simulink model "SUB_LinControl"  (R2018b)
settings: Solver=VariableStepDiscrete  StartTime=0.0  StopTime=10  RelTol=1e-3
PreLoadFcn:
  | if(exist('MBDS_ModelCallback', 'file'))
  |    MBDS_ModelCallback('PreLoad');
  | end
PostLoadFcn:
  | if(exist('MBDS_ModelCallback', 'file'))
  |    MBDS_ModelCallback('PostLoad');
  | end
InitFcn:
  | if(exist('MBDS_ModelCallback', 'file'))
  |    MBDS_ModelCallback('Init');
  | end
StartFcn:
  | if(exist('MBDS_ModelCallback', 'file'))
  |    MBDS_ModelCallback('Start');
  | end
StopFcn:
  | if(exist('MBDS_ModelCallback', 'file'))
  |    MBDS_ModelCallback('Stop');
  | end
undefined symbols (not defined in the file): sigbuilder_block
libraries: KIBES_Signal x48, simulink x3
(part 2 of 2)

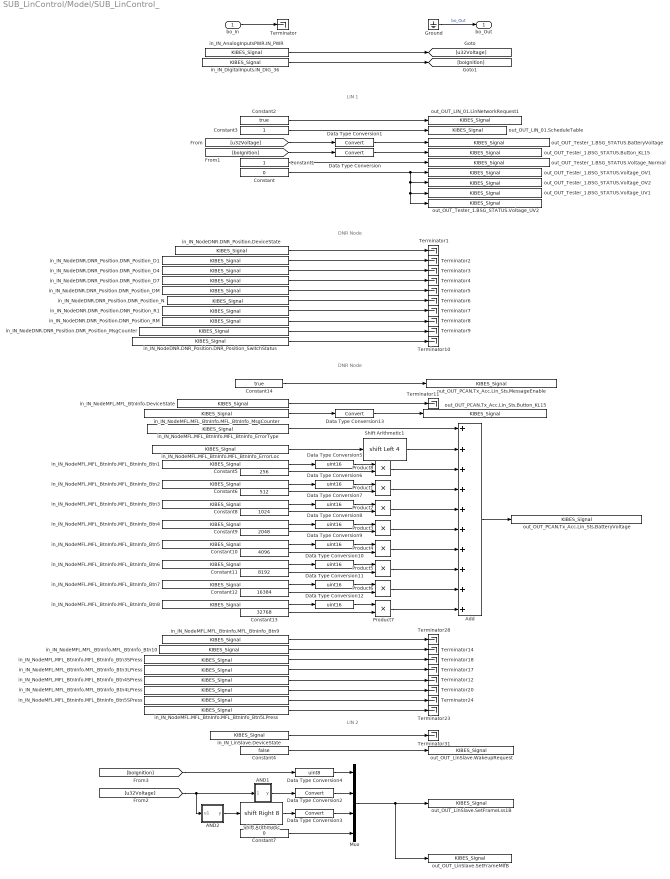
== system SUB_LinControl/Model/SUB_LinControl_ ==
  note: LIN 1
  note: DNR Node
  note: DNR Node
  note: LIN 2
  bo_In : Inport  OutDataTypeStr=boolean
  AND1 : Subsystem  InitFcn=|  mask(AND){MBDS_LibraryBlock=on, BitwiseMode=on, Inputs=1, UseBitMask=on, BitMask='FF', OutDataTypeStr=Inherit: Inherit via back propagation, MBDS_BlockVersion=08.20.02}
      | if(exist('MBDS_BlockCallback', 'file'))
      |    MBDS_BlockCallback('Update', gcb);
      | end
      mask prompts: MBDS_LibraryBlock "MBDS library block"; BitwiseMode "Use 'bitwise' mode"; Inputs "Number of input ports:"; UseBitMask "Use bit mask"; BitMask "Bit mask:"; OutDataTypeStr "Output data type:"; MBDS_BlockVersion "Version:"
      mask help: Logical or bitwise AND operator. For multiple inputs, operators are applied across the inputs. For a single input, operators are applied across the input vector. In bitwise mode a bit mask can be applied onto single input signals.
      mask init:
      | if(exist('MBDS_BlockCallback', 'file'))
      |    MBDS_BlockCallback('Init', gcb);
      | else
      |    % Disable all mask parameters
      |    MaskEnables = get_param(gcb, 'MaskEnables');
      |    for k = [1:length(MaskEnables)]
      |       MaskEnables{k} = 'off';
      |    end
      |    if(~isequal(MaskEnables, get_param(gcb, 'MaskEnables')))
      |       set_param(gcb, 'MaskEnables', MaskEnables);
      |    end
      | end
      settings: AttributesFormatString=bitwise
      mask Help: eval(['open([workdir(''library_dir:''),''\Blockset\help\'',get_param(gcb,''MaskType''),''.html''])'])
      mask Callback BitwiseMode:
      | if(exist('MBDS_BlockCallback', 'file'))
      |    MBDS_BlockCallback('BitwiseMode', gcb);
      | end
      mask Callback Inputs:
      | if(exist('MBDS_BlockCallback', 'file'))
      |    MBDS_BlockCallback('Inputs', gcb);
      | end
      mask Callback UseBitMask:
      | if(exist('MBDS_BlockCallback', 'file'))
      |    MBDS_BlockCallback('UseBitMask', gcb);
      | end
      mask Callback BitMask:
      | if(exist('MBDS_BlockCallback', 'file'))
      |    MBDS_BlockCallback('BitMask', gcb);
      | end
      mask TypeOptions OutDataTypeStr: Inherit: Inherit via back propagation | int8 | uint8 | int16 | uint16 | int32 | uint32 | boolean
      mask Callback OutDataTypeStr:
      | % Adopt Value
      | if(exist('MBDS_BlockCallback', 'file'))
      |    MBDS_BlockCallback('OutDataTypeStr', gcb);
      | end
      mask DialogControl ParameterTabVar0 Prompt: Main
      mask DialogControl ParameterTabVar01 Prompt: Signal Attributes
      mask DialogControl ParameterTabVar012 Prompt: Version
      mask Display:
      | % Show icon or block text
      | if(UseBitMask)
      |    if(isnumeric(BitMask))
      |       BitMaskString = ['0x',dec2hex(floor(BitMask))];
      |    elseif(ischar(BitMask))
      |       BitMaskString = ['0x',upper(BitMask)];
      |    else
      |       BitMaskString = '???';
      |    end
      |    disp(sprintf(['AND\n', BitMaskString]))
      | else
      |    disp('AND')
      | end
  AND2 : Subsystem  InitFcn=|  mask(AND){MBDS_LibraryBlock=on, BitwiseMode=on, Inputs=1, UseBitMask=on, BitMask='FF00', OutDataTypeStr=Inherit: Inherit via back propagation, MBDS_BlockVersion=08.20.02}
      | if(exist('MBDS_BlockCallback', 'file'))
      |    MBDS_BlockCallback('Update', gcb);
      | end
      mask prompts: MBDS_LibraryBlock "MBDS library block"; BitwiseMode "Use 'bitwise' mode"; Inputs "Number of input ports:"; UseBitMask "Use bit mask"; BitMask "Bit mask:"; OutDataTypeStr "Output data type:"; MBDS_BlockVersion "Version:"
      mask help: Logical or bitwise AND operator. For multiple inputs, operators are applied across the inputs. For a single input, operators are applied across the input vector. In bitwise mode a bit mask can be applied onto single input signals.
      mask init: same as SUB_LinControl/Model/SUB_LinControl_/AND1
      settings: AttributesFormatString=bitwise
      mask Help: eval(['open([workdir(''library_dir:''),''\Blockset\help\'',get_param(gcb,''MaskType''),''.html''])'])
      mask Callback BitwiseMode:
      | if(exist('MBDS_BlockCallback', 'file'))
      |    MBDS_BlockCallback('BitwiseMode', gcb);
      | end
      mask Callback Inputs:
      | if(exist('MBDS_BlockCallback', 'file'))
      |    MBDS_BlockCallback('Inputs', gcb);
      | end
      mask Callback UseBitMask:
      | if(exist('MBDS_BlockCallback', 'file'))
      |    MBDS_BlockCallback('UseBitMask', gcb);
      | end
      mask Callback BitMask:
      | if(exist('MBDS_BlockCallback', 'file'))
      |    MBDS_BlockCallback('BitMask', gcb);
      | end
      mask TypeOptions OutDataTypeStr: Inherit: Inherit via back propagation | int8 | uint8 | int16 | uint16 | int32 | uint32 | boolean
      mask Callback OutDataTypeStr:
      | % Adopt Value
      | if(exist('MBDS_BlockCallback', 'file'))
      |    MBDS_BlockCallback('OutDataTypeStr', gcb);
      | end
      mask DialogControl ParameterTabVar0 Prompt: Main
      mask DialogControl ParameterTabVar01 Prompt: Signal Attributes
      mask DialogControl ParameterTabVar012 Prompt: Version
      mask Display:
      | % Show icon or block text
      | if(UseBitMask)
      |    if(isnumeric(BitMask))
      |       BitMaskString = ['0x',dec2hex(floor(BitMask))];
      |    elseif(ischar(BitMask))
      |       BitMaskString = ['0x',upper(BitMask)];
      |    else
      |       BitMaskString = '???';
      |    end
      |    disp(sprintf(['AND\n', BitMaskString]))
      | else
      |    disp('AND')
      | end
  Add : Sum  InitFcn=|  Inputs=++++++++++  AccumDataTypeStr=uint16  OutDataTypeStr=uint16  SaturateOnIntegerOverflow=on
      | if(exist('MBDS_BlockCallback', 'file'))
      |    MBDS_BlockCallback('Update', gcb);  
      | end
      settings: AttributesFormatString=Saturate: %<SaturateOnIntegerOverflow>
  Constant : Constant  InitFcn=|  Value=0  OutDataTypeStr=uint8
      | if(exist('MBDS_BlockCallback', 'file'))
      |    MBDS_BlockCallback('Update', gcb);  
      | end
  Constant1 : Constant  InitFcn=|  OutDataTypeStr=uint8
      | if(exist('MBDS_BlockCallback', 'file'))
      |    MBDS_BlockCallback('Update', gcb);  
      | end
  Constant10 : Constant  InitFcn=|  Value=4096  OutDataTypeStr=uint16
      | if(exist('MBDS_BlockCallback', 'file'))
      |    MBDS_BlockCallback('Update', gcb);  
      | end
  Constant11 : Constant  InitFcn=|  Value=8192  OutDataTypeStr=uint16
      | if(exist('MBDS_BlockCallback', 'file'))
      |    MBDS_BlockCallback('Update', gcb);  
      | end
  Constant12 : Constant  InitFcn=|  Value=16384  OutDataTypeStr=uint16
      | if(exist('MBDS_BlockCallback', 'file'))
      |    MBDS_BlockCallback('Update', gcb);  
      | end
  Constant13 : Constant  InitFcn=|  Value=32768  OutDataTypeStr=uint16
      | if(exist('MBDS_BlockCallback', 'file'))
      |    MBDS_BlockCallback('Update', gcb);  
      | end
  Constant14 : Constant  InitFcn=|  Value=true  OutDataTypeStr=boolean  LockScale=on
      | if(exist('MBDS_BlockCallback', 'file'))
      |    MBDS_BlockCallback('Update', gcb);  
      | end
  Constant2 : Constant  InitFcn=|  Value=true  OutDataTypeStr=boolean
      | if(exist('MBDS_BlockCallback', 'file'))
      |    MBDS_BlockCallback('Update', gcb);  
      | end
  Constant3 : Constant  InitFcn=|  OutDataTypeStr=uint8
      | if(exist('MBDS_BlockCallback', 'file'))
      |    MBDS_BlockCallback('Update', gcb);  
      | end
  Constant4 : Constant  InitFcn=|  Value=false  OutDataTypeStr=boolean
      | if(exist('MBDS_BlockCallback', 'file'))
      |    MBDS_BlockCallback('Update', gcb);  
      | end
  Constant5 : Constant  InitFcn=|  Value=256  OutDataTypeStr=uint16
      | if(exist('MBDS_BlockCallback', 'file'))
      |    MBDS_BlockCallback('Update', gcb);  
      | end
  Constant6 : Constant  InitFcn=|  Value=512  OutDataTypeStr=uint16
      | if(exist('MBDS_BlockCallback', 'file'))
      |    MBDS_BlockCallback('Update', gcb);  
      | end
  Constant7 : Constant  InitFcn=|  Value=0  OutDataTypeStr=uint8
      | if(exist('MBDS_BlockCallback', 'file'))
      |    MBDS_BlockCallback('Update', gcb);  
      | end
  Constant8 : Constant  InitFcn=|  Value=1024  OutDataTypeStr=uint16
      | if(exist('MBDS_BlockCallback', 'file'))
      |    MBDS_BlockCallback('Update', gcb);  
      | end
  Constant9 : Constant  InitFcn=|  Value=2048  OutDataTypeStr=uint16
      | if(exist('MBDS_BlockCallback', 'file'))
      |    MBDS_BlockCallback('Update', gcb);  
      | end
  Data Type Conversion : DataTypeConversion  InitFcn=|  SaturateOnIntegerOverflow=on
      | try
      |    MBDS_BlockCallback('Update', gcb);
      | end
      settings: AttributesFormatString=Saturate: %<SaturateOnIntegerOverflow>
  Data Type Conversion1 : DataTypeConversion  InitFcn=|  SaturateOnIntegerOverflow=on
      | try
      |    MBDS_BlockCallback('Update', gcb);
      | end
      settings: AttributesFormatString=Saturate: %<SaturateOnIntegerOverflow>
  Data Type Conversion10 : DataTypeConversion  InitFcn=|  OutDataTypeStr=uint16  SaturateOnIntegerOverflow=on
      | try
      |    MBDS_BlockCallback('Update', gcb);
      | end
      settings: AttributesFormatString=Saturate: %<SaturateOnIntegerOverflow>
  Data Type Conversion11 : DataTypeConversion  InitFcn=|  OutDataTypeStr=uint16  SaturateOnIntegerOverflow=on
      | try
      |    MBDS_BlockCallback('Update', gcb);
      | end
      settings: AttributesFormatString=Saturate: %<SaturateOnIntegerOverflow>
  Data Type Conversion12 : DataTypeConversion  InitFcn=|  OutDataTypeStr=uint16  SaturateOnIntegerOverflow=on
      | try
      |    MBDS_BlockCallback('Update', gcb);
      | end
      settings: AttributesFormatString=Saturate: %<SaturateOnIntegerOverflow>
  Data Type Conversion13 : DataTypeConversion  InitFcn=|  SaturateOnIntegerOverflow=on
      | try
      |    MBDS_BlockCallback('Update', gcb);
      | end
      settings: AttributesFormatString=Saturate: %<SaturateOnIntegerOverflow>
  Data Type Conversion2 : DataTypeConversion  InitFcn=|
      | try
      |    MBDS_BlockCallback('Update', gcb);
      | end
      settings: AttributesFormatString=Saturate: %<SaturateOnIntegerOverflow>
  Data Type Conversion3 : DataTypeConversion  InitFcn=|
      | try
      |    MBDS_BlockCallback('Update', gcb);
      | end
      settings: AttributesFormatString=Saturate: %<SaturateOnIntegerOverflow>
  Data Type Conversion4 : DataTypeConversion  InitFcn=|  OutDataTypeStr=uint8  SaturateOnIntegerOverflow=on
      | try
      |    MBDS_BlockCallback('Update', gcb);
      | end
      settings: AttributesFormatString=Saturate: %<SaturateOnIntegerOverflow>
  Data Type Conversion5 : DataTypeConversion  InitFcn=|  OutDataTypeStr=uint16  SaturateOnIntegerOverflow=on
      | try
      |    MBDS_BlockCallback('Update', gcb);
      | end
      settings: AttributesFormatString=Saturate: %<SaturateOnIntegerOverflow>
  Data Type Conversion6 : DataTypeConversion  InitFcn=|  OutDataTypeStr=uint16  SaturateOnIntegerOverflow=on
      | try
      |    MBDS_BlockCallback('Update', gcb);
      | end
      settings: AttributesFormatString=Saturate: %<SaturateOnIntegerOverflow>
  Data Type Conversion7 : DataTypeConversion  InitFcn=|  OutDataTypeStr=uint16  SaturateOnIntegerOverflow=on
      | try
      |    MBDS_BlockCallback('Update', gcb);
      | end
      settings: AttributesFormatString=Saturate: %<SaturateOnIntegerOverflow>
  Data Type Conversion8 : DataTypeConversion  InitFcn=|  OutDataTypeStr=uint16  SaturateOnIntegerOverflow=on
      | try
      |    MBDS_BlockCallback('Update', gcb);
      | end
      settings: AttributesFormatString=Saturate: %<SaturateOnIntegerOverflow>
  Data Type Conversion9 : DataTypeConversion  InitFcn=|  OutDataTypeStr=uint16  SaturateOnIntegerOverflow=on
      | try
      |    MBDS_BlockCallback('Update', gcb);
      | end
      settings: AttributesFormatString=Saturate: %<SaturateOnIntegerOverflow>
  Ground : Ground  InitFcn=|
      | try
      |    MBDS_BlockCallback('Update', gcb);
      | end
      settings: MoveFcn=UpdateBlockSize(gcb);
  Mux : Mux  InitFcn=|
      | try
      |    MBDS_BlockCallback('Update', gcb);
      | end
  Product1 : Product  InitFcn=|  Inputs=**  OutDataTypeStr=uint16  SaturateOnIntegerOverflow=on
      | if(exist('MBDS_BlockCallback', 'file'))
      |    MBDS_BlockCallback('Update', gcb);  
      | end
      settings: AttributesFormatString=Saturate: %<SaturateOnIntegerOverflow>
  Product2 : Product  InitFcn=|  Inputs=**  OutDataTypeStr=uint16  SaturateOnIntegerOverflow=on
      | if(exist('MBDS_BlockCallback', 'file'))
      |    MBDS_BlockCallback('Update', gcb);  
      | end
      settings: AttributesFormatString=Saturate: %<SaturateOnIntegerOverflow>
  Product3 : Product  InitFcn=|  Inputs=**  OutDataTypeStr=uint16  SaturateOnIntegerOverflow=on
      | if(exist('MBDS_BlockCallback', 'file'))
      |    MBDS_BlockCallback('Update', gcb);  
      | end
      settings: AttributesFormatString=Saturate: %<SaturateOnIntegerOverflow>
  Product4 : Product  InitFcn=|  Inputs=**  OutDataTypeStr=uint16  SaturateOnIntegerOverflow=on
      | if(exist('MBDS_BlockCallback', 'file'))
      |    MBDS_BlockCallback('Update', gcb);  
      | end
      settings: AttributesFormatString=Saturate: %<SaturateOnIntegerOverflow>
  Product5 : Product  InitFcn=|  Inputs=**  OutDataTypeStr=uint16  SaturateOnIntegerOverflow=on
      | if(exist('MBDS_BlockCallback', 'file'))
      |    MBDS_BlockCallback('Update', gcb);  
      | end
      settings: AttributesFormatString=Saturate: %<SaturateOnIntegerOverflow>
  Product6 : Product  InitFcn=|  Inputs=**  OutDataTypeStr=uint16  SaturateOnIntegerOverflow=on
      | if(exist('MBDS_BlockCallback', 'file'))
      |    MBDS_BlockCallback('Update', gcb);  
      | end
      settings: AttributesFormatString=Saturate: %<SaturateOnIntegerOverflow>
  Product7 : Product  InitFcn=|  Inputs=**  OutDataTypeStr=uint16  SaturateOnIntegerOverflow=on
      | if(exist('MBDS_BlockCallback', 'file'))
      |    MBDS_BlockCallback('Update', gcb);  
      | end
      settings: AttributesFormatString=Saturate: %<SaturateOnIntegerOverflow>
  Product8 : Product  InitFcn=|  Inputs=**  OutDataTypeStr=uint16  SaturateOnIntegerOverflow=on
      | if(exist('MBDS_BlockCallback', 'file'))
      |    MBDS_BlockCallback('Update', gcb);  
      | end
      settings: AttributesFormatString=Saturate: %<SaturateOnIntegerOverflow>
  Shift Arithmetic : ArithShift  InitFcn=|  BitShiftNumber=8  BitShiftDirection=Right
      | try
      |    MBDS_BlockCallback('Update', gcb);
      | end
  Shift Arithmetic1 : ArithShift  InitFcn=|  BitShiftNumber=4  BitShiftDirection=Left
      | try
      |    MBDS_BlockCallback('Update', gcb);
      | end
  Terminator{,1..12,14,17..18,20,23..24,28,31} (21 alike) : Terminator
      settings: MoveFcn=UpdateBlockSize(gcb);
      settings: InitFcn=|
      | try
      |    MBDS_BlockCallback('Update', gcb);
      | end
  in_IN_AnalogInputsPWR.IN_PWR : KIBES_Signal/KIBES_Signal  MBDS_LibraryBlock=on  DatabaseKey=721  SignalName=IN_AnalogInputsPWR.IN_PWR  SymbolName=IN_AnalogInputsPWR_IN_PWR_000721  DataType=uint32  Init=0  Slope=1  Bias=0  DataSize=1  fpDataType=uint32  BlockIOType=Inport  DeviceType=0
  in_IN_DigitalInputs.IN_DIG_36 : KIBES_Signal/KIBES_Signal  MBDS_LibraryBlock=on  DatabaseKey=60  SignalName=IN_DigitalInputs.IN_DIG_36  SymbolName=IN_DigitalInputs_IN_DIG_36_000060  DataType=boolean  Init=0  Slope=1  Bias=0  DataSize=1  fpDataType=boolean  BlockIOType=Inport  DeviceType=0
  in_IN_LinSlave.DeviceState : KIBES_Signal/KIBES_Signal  MBDS_LibraryBlock=on  DatabaseKey=2325  SignalName=IN_LinSlave.DeviceState  SymbolName=IN_LinSlave_DeviceState_002325  DataType=uint16  Init=0  Slope=1  Bias=0  DataSize=1  fpDataType=uint16  BlockIOType=Inport  DeviceType=0
  in_IN_NodeDNR.DNR_Position.DNR_Position_D1 : KIBES_Signal/KIBES_Signal  MBDS_LibraryBlock=on  DatabaseKey=1352  SignalName=IN_NodeDNR.DNR_Position.DNR_Position_D1  SymbolName=IN_NodeDNR_DNR_Position_DNR_Position_D1_001352  DataType=uint8  Init=0  Slope=1  Bias=0  DataSize=1  fpDataType=uint8  BlockIOType=Inport  DeviceType=0
  in_IN_NodeDNR.DNR_Position.DNR_Position_D4 : KIBES_Signal/KIBES_Signal  MBDS_LibraryBlock=on  DatabaseKey=1353  SignalName=IN_NodeDNR.DNR_Position.DNR_Position_D4  SymbolName=IN_NodeDNR_DNR_Position_DNR_Position_D4_001353  DataType=uint8  Init=0  Slope=1  Bias=0  DataSize=1  fpDataType=uint8  BlockIOType=Inport  DeviceType=0
  in_IN_NodeDNR.DNR_Position.DNR_Position_D7 : KIBES_Signal/KIBES_Signal  MBDS_LibraryBlock=on  DatabaseKey=1354  SignalName=IN_NodeDNR.DNR_Position.DNR_Position_D7  SymbolName=IN_NodeDNR_DNR_Position_DNR_Position_D7_001354  DataType=uint8  Init=0  Slope=1  Bias=0  DataSize=1  fpDataType=uint8  BlockIOType=Inport  DeviceType=0
  in_IN_NodeDNR.DNR_Position.DNR_Position_DM : KIBES_Signal/KIBES_Signal  MBDS_LibraryBlock=on  DatabaseKey=1355  SignalName=IN_NodeDNR.DNR_Position.DNR_Position_DM  SymbolName=IN_NodeDNR_DNR_Position_DNR_Position_DM_001355  DataType=uint8  Init=0  Slope=1  Bias=0  DataSize=1  fpDataType=uint8  BlockIOType=Inport  DeviceType=0
  in_IN_NodeDNR.DNR_Position.DNR_Position_MsgCounter : KIBES_Signal/KIBES_Signal  MBDS_LibraryBlock=on  DatabaseKey=1356  SignalName=IN_NodeDNR.DNR_Position.DNR_Position_MsgCounter  SymbolName=IN_NodeDNR_DNR_Position_DNR_Position_MsgCounter_001356  DataType=uint8  Init=0  Slope=1  Bias=0  DataSize=1  fpDataType=uint8  BlockIOType=Inport  DeviceType=0
  in_IN_NodeDNR.DNR_Position.DNR_Position_N : KIBES_Signal/KIBES_Signal  MBDS_LibraryBlock=on  DatabaseKey=1351  SignalName=IN_NodeDNR.DNR_Position.DNR_Position_N  SymbolName=IN_NodeDNR_DNR_Position_DNR_Position_N_001351  DataType=uint8  Init=0  Slope=1  Bias=0  DataSize=1  fpDataType=uint8  BlockIOType=Inport  DeviceType=0
  in_IN_NodeDNR.DNR_Position.DNR_Position_R1 : KIBES_Signal/KIBES_Signal  MBDS_LibraryBlock=on  DatabaseKey=1350  SignalName=IN_NodeDNR.DNR_Position.DNR_Position_R1  SymbolName=IN_NodeDNR_DNR_Position_DNR_Position_R1_001350  DataType=uint8  Init=0  Slope=1  Bias=0  DataSize=1  fpDataType=uint8  BlockIOType=Inport  DeviceType=0
  in_IN_NodeDNR.DNR_Position.DNR_Position_RM : KIBES_Signal/KIBES_Signal  MBDS_LibraryBlock=on  DatabaseKey=1349  SignalName=IN_NodeDNR.DNR_Position.DNR_Position_RM  SymbolName=IN_NodeDNR_DNR_Position_DNR_Position_RM_001349  DataType=uint8  Init=0  Slope=1  Bias=0  DataSize=1  fpDataType=uint8  BlockIOType=Inport  DeviceType=0
  in_IN_NodeDNR.DNR_Position.DNR_Position_SwitchStatus : KIBES_Signal/KIBES_Signal  MBDS_LibraryBlock=on  DatabaseKey=1357  SignalName=IN_NodeDNR.DNR_Position.DNR_Position_SwitchStatus  SymbolName=IN_NodeDNR_DNR_Position_DNR_Position_SwitchStatus_001357  DataType=uint8  Init=0  Slope=1  Bias=0  DataSize=1  fpDataType=uint8  BlockIOType=Inport  DeviceType=0
  in_IN_NodeDNR.DNR_Position.DeviceState : KIBES_Signal/KIBES_Signal  MBDS_LibraryBlock=on  DatabaseKey=2273  SignalName=IN_NodeDNR.DNR_Position.DeviceState  SymbolName=IN_NodeDNR_DNR_Position_DeviceState_002273  DataType=uint16  Init=0  Slope=1  Bias=0  DataSize=1  fpDataType=uint16  BlockIOType=Inport  DeviceType=0
  in_IN_NodeMFL.MFL_BtnInfo.DeviceState : KIBES_Signal/KIBES_Signal  MBDS_LibraryBlock=on  DatabaseKey=2272  SignalName=IN_NodeMFL.MFL_BtnInfo.DeviceState  SymbolName=IN_NodeMFL_MFL_BtnInfo_DeviceState_002272  DataType=uint16  Init=0  Slope=1  Bias=0  DataSize=1  fpDataType=uint16  BlockIOType=Inport  DeviceType=0
  in_IN_NodeMFL.MFL_BtnInfo.MFL_BtnInfo_Btn1 : KIBES_Signal/KIBES_Signal  MBDS_LibraryBlock=on  DatabaseKey=1361  SignalName=IN_NodeMFL.MFL_BtnInfo.MFL_BtnInfo_Btn1  SymbolName=IN_NodeMFL_MFL_BtnInfo_MFL_BtnInfo_Btn1_001361  DataType=uint8  Init=0  Slope=1  Bias=0  DataSize=1  fpDataType=uint8  BlockIOType=Inport  DeviceType=0
  in_IN_NodeMFL.MFL_BtnInfo.MFL_BtnInfo_Btn10 : KIBES_Signal/KIBES_Signal  MBDS_LibraryBlock=on  DatabaseKey=1370  SignalName=IN_NodeMFL.MFL_BtnInfo.MFL_BtnInfo_Btn10  SymbolName=IN_NodeMFL_MFL_BtnInfo_MFL_BtnInfo_Btn10_001370  DataType=uint8  Init=0  Slope=1  Bias=0  DataSize=1  fpDataType=uint8  BlockIOType=Inport  DeviceType=0
  in_IN_NodeMFL.MFL_BtnInfo.MFL_BtnInfo_Btn2 : KIBES_Signal/KIBES_Signal  MBDS_LibraryBlock=on  DatabaseKey=1362  SignalName=IN_NodeMFL.MFL_BtnInfo.MFL_BtnInfo_Btn2  SymbolName=IN_NodeMFL_MFL_BtnInfo_MFL_BtnInfo_Btn2_001362  DataType=uint8  Init=0  Slope=1  Bias=0  DataSize=1  fpDataType=uint8  BlockIOType=Inport  DeviceType=0
  in_IN_NodeMFL.MFL_BtnInfo.MFL_BtnInfo_Btn3 : KIBES_Signal/KIBES_Signal  MBDS_LibraryBlock=on  DatabaseKey=1363  SignalName=IN_NodeMFL.MFL_BtnInfo.MFL_BtnInfo_Btn3  SymbolName=IN_NodeMFL_MFL_BtnInfo_MFL_BtnInfo_Btn3_001363  DataType=uint8  Init=0  Slope=1  Bias=0  DataSize=1  fpDataType=uint8  BlockIOType=Inport  DeviceType=0
  in_IN_NodeMFL.MFL_BtnInfo.MFL_BtnInfo_Btn3LPress : KIBES_Signal/KIBES_Signal  MBDS_LibraryBlock=on  DatabaseKey=1372  SignalName=IN_NodeMFL.MFL_BtnInfo.MFL_BtnInfo_Btn3LPress  SymbolName=IN_NodeMFL_MFL_BtnInfo_MFL_BtnInfo_Btn3LPress_001372  DataType=uint8  Init=0  Slope=1  Bias=0  DataSize=1  fpDataType=uint8  BlockIOType=Inport  DeviceType=0
  in_IN_NodeMFL.MFL_BtnInfo.MFL_BtnInfo_Btn3SPress : KIBES_Signal/KIBES_Signal  MBDS_LibraryBlock=on  DatabaseKey=1371  SignalName=IN_NodeMFL.MFL_BtnInfo.MFL_BtnInfo_Btn3SPress  SymbolName=IN_NodeMFL_MFL_BtnInfo_MFL_BtnInfo_Btn3SPress_001371  DataType=uint8  Init=0  Slope=1  Bias=0  DataSize=1  fpDataType=uint8  BlockIOType=Inport  DeviceType=0
  in_IN_NodeMFL.MFL_BtnInfo.MFL_BtnInfo_Btn4 : KIBES_Signal/KIBES_Signal  MBDS_LibraryBlock=on  DatabaseKey=1364  SignalName=IN_NodeMFL.MFL_BtnInfo.MFL_BtnInfo_Btn4  SymbolName=IN_NodeMFL_MFL_BtnInfo_MFL_BtnInfo_Btn4_001364  DataType=uint8  Init=0  Slope=1  Bias=0  DataSize=1  fpDataType=uint8  BlockIOType=Inport  DeviceType=0
  in_IN_NodeMFL.MFL_BtnInfo.MFL_BtnInfo_Btn4LPress : KIBES_Signal/KIBES_Signal  MBDS_LibraryBlock=on  DatabaseKey=1374  SignalName=IN_NodeMFL.MFL_BtnInfo.MFL_BtnInfo_Btn4LPress  SymbolName=IN_NodeMFL_MFL_BtnInfo_MFL_BtnInfo_Btn4LPress_001374  DataType=uint8  Init=0  Slope=1  Bias=0  DataSize=1  fpDataType=uint8  BlockIOType=Inport  DeviceType=0
  in_IN_NodeMFL.MFL_BtnInfo.MFL_BtnInfo_Btn4SPress : KIBES_Signal/KIBES_Signal  MBDS_LibraryBlock=on  DatabaseKey=1373  SignalName=IN_NodeMFL.MFL_BtnInfo.MFL_BtnInfo_Btn4SPress  SymbolName=IN_NodeMFL_MFL_BtnInfo_MFL_BtnInfo_Btn4SPress_001373  DataType=uint8  Init=0  Slope=1  Bias=0  DataSize=1  fpDataType=uint8  BlockIOType=Inport  DeviceType=0
  in_IN_NodeMFL.MFL_BtnInfo.MFL_BtnInfo_Btn5 : KIBES_Signal/KIBES_Signal  MBDS_LibraryBlock=on  DatabaseKey=1365  SignalName=IN_NodeMFL.MFL_BtnInfo.MFL_BtnInfo_Btn5  SymbolName=IN_NodeMFL_MFL_BtnInfo_MFL_BtnInfo_Btn5_001365  DataType=uint8  Init=0  Slope=1  Bias=0  DataSize=1  fpDataType=uint8  BlockIOType=Inport  DeviceType=0
  in_IN_NodeMFL.MFL_BtnInfo.MFL_BtnInfo_Btn5LPress : KIBES_Signal/KIBES_Signal  MBDS_LibraryBlock=on  DatabaseKey=1376  SignalName=IN_NodeMFL.MFL_BtnInfo.MFL_BtnInfo_Btn5LPress  SymbolName=IN_NodeMFL_MFL_BtnInfo_MFL_BtnInfo_Btn5LPress_001376  DataType=uint8  Init=0  Slope=1  Bias=0  DataSize=1  fpDataType=uint8  BlockIOType=Inport  DeviceType=0
  in_IN_NodeMFL.MFL_BtnInfo.MFL_BtnInfo_Btn5SPress : KIBES_Signal/KIBES_Signal  MBDS_LibraryBlock=on  DatabaseKey=1375  SignalName=IN_NodeMFL.MFL_BtnInfo.MFL_BtnInfo_Btn5SPress  SymbolName=IN_NodeMFL_MFL_BtnInfo_MFL_BtnInfo_Btn5SPress_001375  DataType=uint8  Init=0  Slope=1  Bias=0  DataSize=1  fpDataType=uint8  BlockIOType=Inport  DeviceType=0
  in_IN_NodeMFL.MFL_BtnInfo.MFL_BtnInfo_Btn6 : KIBES_Signal/KIBES_Signal  MBDS_LibraryBlock=on  DatabaseKey=1366  SignalName=IN_NodeMFL.MFL_BtnInfo.MFL_BtnInfo_Btn6  SymbolName=IN_NodeMFL_MFL_BtnInfo_MFL_BtnInfo_Btn6_001366  DataType=uint8  Init=0  Slope=1  Bias=0  DataSize=1  fpDataType=uint8  BlockIOType=Inport  DeviceType=0
  in_IN_NodeMFL.MFL_BtnInfo.MFL_BtnInfo_Btn7 : KIBES_Signal/KIBES_Signal  MBDS_LibraryBlock=on  DatabaseKey=1367  SignalName=IN_NodeMFL.MFL_BtnInfo.MFL_BtnInfo_Btn7  SymbolName=IN_NodeMFL_MFL_BtnInfo_MFL_BtnInfo_Btn7_001367  DataType=uint8  Init=0  Slope=1  Bias=0  DataSize=1  fpDataType=uint8  BlockIOType=Inport  DeviceType=0
  in_IN_NodeMFL.MFL_BtnInfo.MFL_BtnInfo_Btn8 : KIBES_Signal/KIBES_Signal  MBDS_LibraryBlock=on  DatabaseKey=1368  SignalName=IN_NodeMFL.MFL_BtnInfo.MFL_BtnInfo_Btn8  SymbolName=IN_NodeMFL_MFL_BtnInfo_MFL_BtnInfo_Btn8_001368  DataType=uint8  Init=0  Slope=1  Bias=0  DataSize=1  fpDataType=uint8  BlockIOType=Inport  DeviceType=0
  in_IN_NodeMFL.MFL_BtnInfo.MFL_BtnInfo_Btn9 : KIBES_Signal/KIBES_Signal  MBDS_LibraryBlock=on  DatabaseKey=1369  SignalName=IN_NodeMFL.MFL_BtnInfo.MFL_BtnInfo_Btn9  SymbolName=IN_NodeMFL_MFL_BtnInfo_MFL_BtnInfo_Btn9_001369  DataType=uint8  Init=0  Slope=1  Bias=0  DataSize=1  fpDataType=uint8  BlockIOType=Inport  DeviceType=0
  in_IN_NodeMFL.MFL_BtnInfo.MFL_BtnInfo_ErrorLoc : KIBES_Signal/KIBES_Signal  MBDS_LibraryBlock=on  DatabaseKey=1360  SignalName=IN_NodeMFL.MFL_BtnInfo.MFL_BtnInfo_ErrorLoc  SymbolName=IN_NodeMFL_MFL_BtnInfo_MFL_BtnInfo_ErrorLoc_001360  DataType=uint8  Init=0  Slope=1  Bias=0  DataSize=1  fpDataType=uint8  BlockIOType=Inport  DeviceType=0
  in_IN_NodeMFL.MFL_BtnInfo.MFL_BtnInfo_ErrorType : KIBES_Signal/KIBES_Signal  MBDS_LibraryBlock=on  DatabaseKey=1359  SignalName=IN_NodeMFL.MFL_BtnInfo.MFL_BtnInfo_ErrorType  SymbolName=IN_NodeMFL_MFL_BtnInfo_MFL_BtnInfo_ErrorType_001359  DataType=uint8  Init=0  Slope=1  Bias=0  DataSize=1  fpDataType=uint8  BlockIOType=Inport  DeviceType=0
  in_IN_NodeMFL.MFL_BtnInfo.MFL_BtnInfo_MsgCounter : KIBES_Signal/KIBES_Signal  MBDS_LibraryBlock=on  DatabaseKey=1358  SignalName=IN_NodeMFL.MFL_BtnInfo.MFL_BtnInfo_MsgCounter  SymbolName=IN_NodeMFL_MFL_BtnInfo_MFL_BtnInfo_MsgCounter_001358  DataType=uint8  Init=0  Slope=1  Bias=0  DataSize=1  fpDataType=uint8  BlockIOType=Inport  DeviceType=0
  out_OUT_LIN_01.LinNetworkRequest1 : KIBES_Signal/KIBES_Signal  MBDS_LibraryBlock=on  DatabaseKey=1396  SignalName=OUT_LIN_01.LinNetworkRequest1  SymbolName=OUT_LIN_01_LinNetworkRequest1_001396  DataType=boolean  Init=0  Slope=1  Bias=0  DataSize=1  fpDataType=boolean  BlockIOType=Outport  DeviceType=0
  out_OUT_LIN_01.ScheduleTable : KIBES_Signal/KIBES_Signal  MBDS_LibraryBlock=on  DatabaseKey=1397  SignalName=OUT_LIN_01.ScheduleTable  SymbolName=OUT_LIN_01_ScheduleTable_001397  DataType=uint8  Init=0  Slope=1  Bias=0  DataSize=1  fpDataType=uint8  BlockIOType=Outport  DeviceType=0
  out_OUT_LinSlave.SetFrameLss1B : KIBES_Signal/KIBES_Signal  MBDS_LibraryBlock=on  DatabaseKey=2326  SignalName=OUT_LinSlave.SetFrameLss1B  SymbolName=OUT_LinSlave_SetFrameLss1B_002326  DataType=uint8  Init=[0 0 0 0]  Slope=1  Bias=0  DataSize=4  fpDataType=uint8  BlockIOType=Outport  DeviceType=0
  out_OUT_LinSlave.SetFrameMlfB : KIBES_Signal/KIBES_Signal  MBDS_LibraryBlock=on  DatabaseKey=2327  SignalName=OUT_LinSlave.SetFrameMlfB  SymbolName=OUT_LinSlave_SetFrameMlfB_002327  DataType=uint8  Init=[0 0 0 0]  Slope=1  Bias=0  DataSize=4  fpDataType=uint8  BlockIOType=Outport  DeviceType=0
  out_OUT_LinSlave.WakeupRequest : KIBES_Signal/KIBES_Signal  MBDS_LibraryBlock=on  DatabaseKey=2328  SignalName=OUT_LinSlave.WakeupRequest  SymbolName=OUT_LinSlave_WakeupRequest_002328  DataType=boolean  Init=0  Slope=1  Bias=0  DataSize=1  fpDataType=boolean  BlockIOType=Outport  DeviceType=0
  out_OUT_PCAN.Tx_Acc.Lin_Sts.BatteryVoltage : KIBES_Signal/KIBES_Signal  MBDS_LibraryBlock=on  DatabaseKey=1647  SignalName=OUT_PCAN.Tx_Acc.Lin_Sts.BatteryVoltage  SymbolName=OUT_PCAN_Tx_Acc_Lin_Sts_BatteryVoltage_001647  DataType=uint16  Init=0  Slope=1  Bias=0  DataSize=1  fpDataType=uint16  BlockIOType=Outport  DeviceType=0
  out_OUT_PCAN.Tx_Acc.Lin_Sts.Button_KL15 : KIBES_Signal/KIBES_Signal  MBDS_LibraryBlock=on  DatabaseKey=1648  SignalName=OUT_PCAN.Tx_Acc.Lin_Sts.Button_KL15  SymbolName=OUT_PCAN_Tx_Acc_Lin_Sts_Button_KL15_001648  DataType=boolean  Init=0  Slope=1  Bias=0  DataSize=1  fpDataType=boolean  BlockIOType=Outport  DeviceType=0
  out_OUT_PCAN.Tx_Acc.Lin_Sts.MessageEnable : KIBES_Signal/KIBES_Signal  MBDS_LibraryBlock=on  DatabaseKey=1677  SignalName=OUT_PCAN.Tx_Acc.Lin_Sts.MessageEnable  SymbolName=OUT_PCAN_Tx_Acc_Lin_Sts_MessageEnable_001677  DataType=boolean  Init=0  Slope=1  Bias=0  DataSize=1  fpDataType=boolean  BlockIOType=Outport  DeviceType=0
  out_OUT_Tester_1.BSG_STATUS.BatteryVoltage : KIBES_Signal/KIBES_Signal  MBDS_LibraryBlock=on  DatabaseKey=1395  SignalName=OUT_Tester_1.BSG_STATUS.BatteryVoltage  SymbolName=OUT_Tester_1_BSG_STATUS_BatteryVoltage_001395  DataType=uint16  Init=0  Slope=1  Bias=0  DataSize=1  fpDataType=uint16  BlockIOType=Outport  DeviceType=0
  out_OUT_Tester_1.BSG_STATUS.Button_KL15 : KIBES_Signal/KIBES_Signal  MBDS_LibraryBlock=on  DatabaseKey=1389  SignalName=OUT_Tester_1.BSG_STATUS.Button_KL15  SymbolName=OUT_Tester_1_BSG_STATUS_Button_KL15_001389  DataType=uint8  Init=0  Slope=1  Bias=0  DataSize=1  fpDataType=uint8  BlockIOType=Outport  DeviceType=0
  out_OUT_Tester_1.BSG_STATUS.Voltage_Normal : KIBES_Signal/KIBES_Signal  MBDS_LibraryBlock=on  DatabaseKey=1390  SignalName=OUT_Tester_1.BSG_STATUS.Voltage_Normal  SymbolName=OUT_Tester_1_BSG_STATUS_Voltage_Normal_001390  DataType=uint8  Init=0  Slope=1  Bias=0  DataSize=1  fpDataType=uint8  BlockIOType=Outport  DeviceType=0
  out_OUT_Tester_1.BSG_STATUS.Voltage_OV1 : KIBES_Signal/KIBES_Signal  MBDS_LibraryBlock=on  DatabaseKey=1391  SignalName=OUT_Tester_1.BSG_STATUS.Voltage_OV1  SymbolName=OUT_Tester_1_BSG_STATUS_Voltage_OV1_001391  DataType=uint8  Init=0  Slope=1  Bias=0  DataSize=1  fpDataType=uint8  BlockIOType=Outport  DeviceType=0
  out_OUT_Tester_1.BSG_STATUS.Voltage_OV2 : KIBES_Signal/KIBES_Signal  MBDS_LibraryBlock=on  DatabaseKey=1392  SignalName=OUT_Tester_1.BSG_STATUS.Voltage_OV2  SymbolName=OUT_Tester_1_BSG_STATUS_Voltage_OV2_001392  DataType=uint8  Init=0  Slope=1  Bias=0  DataSize=1  fpDataType=uint8  BlockIOType=Outport  DeviceType=0
  out_OUT_Tester_1.BSG_STATUS.Voltage_UV1 : KIBES_Signal/KIBES_Signal  MBDS_LibraryBlock=on  DatabaseKey=1393  SignalName=OUT_Tester_1.BSG_STATUS.Voltage_UV1  SymbolName=OUT_Tester_1_BSG_STATUS_Voltage_UV1_001393  DataType=uint8  Init=0  Slope=1  Bias=0  DataSize=1  fpDataType=uint8  BlockIOType=Outport  DeviceType=0
  out_OUT_Tester_1.BSG_STATUS.Voltage_UV2 : KIBES_Signal/KIBES_Signal  MBDS_LibraryBlock=on  DatabaseKey=1394  SignalName=OUT_Tester_1.BSG_STATUS.Voltage_UV2  SymbolName=OUT_Tester_1_BSG_STATUS_Voltage_UV2_001394  DataType=uint8  Init=0  Slope=1  Bias=0  DataSize=1  fpDataType=uint8  BlockIOType=Outport  DeviceType=0
  bo_Out : Outport  OutDataTypeStr=boolean
  wires:
  bo_In/1 -> Terminator/1
  Ground/1 -> bo_Out/1  "bo_Out"
  Constant/1 -> out_OUT_Tester_1.BSG_STATUS.Voltage_UV2/1, out_OUT_Tester_1.BSG_STATUS.Voltage_UV1/1, out_OUT_Tester_1.BSG_STATUS.Voltage_OV2/1, out_OUT_Tester_1.BSG_STATUS.Voltage_OV1/1
  Constant1/1 -> out_OUT_Tester_1.BSG_STATUS.Voltage_Normal/1
  [boIgnition] -> Data Type Conversion/1
  Data Type Conversion/1 -> out_OUT_Tester_1.BSG_STATUS.Button_KL15/1
  [u32Voltage] -> Data Type Conversion1/1
  Data Type Conversion1/1 -> out_OUT_Tester_1.BSG_STATUS.BatteryVoltage/1
  Constant2/1 -> out_OUT_LIN_01.LinNetworkRequest1/1
  Constant3/1 -> out_OUT_LIN_01.ScheduleTable/1
  in_IN_NodeDNR.DNR_Position.DeviceState/1 -> Terminator1/1
  in_IN_NodeDNR.DNR_Position.DNR_Position_D1/1 -> Terminator2/1
  in_IN_NodeDNR.DNR_Position.DNR_Position_D4/1 -> Terminator3/1
  in_IN_NodeDNR.DNR_Position.DNR_Position_D7/1 -> Terminator4/1
  in_IN_NodeDNR.DNR_Position.DNR_Position_DM/1 -> Terminator5/1
  in_IN_NodeDNR.DNR_Position.DNR_Position_N/1 -> Terminator6/1
  in_IN_NodeDNR.DNR_Position.DNR_Position_R1/1 -> Terminator7/1
  in_IN_NodeDNR.DNR_Position.DNR_Position_RM/1 -> Terminator8/1
  in_IN_NodeDNR.DNR_Position.DNR_Position_MsgCounter/1 -> Terminator9/1
  in_IN_NodeDNR.DNR_Position.DNR_Position_SwitchStatus/1 -> Terminator10/1
  in_IN_NodeMFL.MFL_BtnInfo.DeviceState/1 -> Terminator11/1
  in_IN_NodeMFL.MFL_BtnInfo.MFL_BtnInfo_Btn1/1 -> Data Type Conversion5/1
  in_IN_NodeMFL.MFL_BtnInfo.MFL_BtnInfo_Btn10/1 -> Terminator14/1
  in_IN_NodeMFL.MFL_BtnInfo.MFL_BtnInfo_Btn2/1 -> Data Type Conversion6/1
  in_IN_NodeMFL.MFL_BtnInfo.MFL_BtnInfo_Btn3/1 -> Data Type Conversion7/1
  in_IN_NodeMFL.MFL_BtnInfo.MFL_BtnInfo_Btn3LPress/1 -> Terminator17/1
  in_IN_NodeMFL.MFL_BtnInfo.MFL_BtnInfo_Btn3SPress/1 -> Terminator18/1
  in_IN_NodeMFL.MFL_BtnInfo.MFL_BtnInfo_Btn4/1 -> Data Type Conversion8/1
  in_IN_NodeMFL.MFL_BtnInfo.MFL_BtnInfo_Btn4LPress/1 -> Terminator20/1
  in_IN_NodeMFL.MFL_BtnInfo.MFL_BtnInfo_Btn4SPress/1 -> Terminator12/1
  in_IN_NodeMFL.MFL_BtnInfo.MFL_BtnInfo_Btn5/1 -> Data Type Conversion9/1
  in_IN_NodeMFL.MFL_BtnInfo.MFL_BtnInfo_Btn5LPress/1 -> Terminator23/1
  in_IN_NodeMFL.MFL_BtnInfo.MFL_BtnInfo_Btn5SPress/1 -> Terminator24/1
  in_IN_NodeMFL.MFL_BtnInfo.MFL_BtnInfo_Btn6/1 -> Data Type Conversion10/1
  in_IN_NodeMFL.MFL_BtnInfo.MFL_BtnInfo_Btn7/1 -> Data Type Conversion11/1
  in_IN_NodeMFL.MFL_BtnInfo.MFL_BtnInfo_Btn8/1 -> Data Type Conversion12/1
  in_IN_NodeMFL.MFL_BtnInfo.MFL_BtnInfo_Btn9/1 -> Terminator28/1
  in_IN_NodeMFL.MFL_BtnInfo.MFL_BtnInfo_ErrorLoc/1 -> Shift Arithmetic1/1
  in_IN_NodeMFL.MFL_BtnInfo.MFL_BtnInfo_ErrorType/1 -> Add/1
  in_IN_NodeMFL.MFL_BtnInfo.MFL_BtnInfo_MsgCounter/1 -> Data Type Conversion13/1
  in_IN_LinSlave.DeviceState/1 -> Terminator31/1
  Constant4/1 -> out_OUT_LinSlave.WakeupRequest/1
  Mux/1 -> out_OUT_LinSlave.SetFrameMlfB/1, out_OUT_LinSlave.SetFrameLss1B/1
  Constant7/1 -> Mux/4
  in_IN_AnalogInputsPWR.IN_PWR/1 -> [u32Voltage]
  in_IN_DigitalInputs.IN_DIG_36/1 -> [boIgnition]
  Data Type Conversion2/1 -> Mux/2
  AND1/1(y) -> Data Type Conversion2/1
  [u32Voltage] -> AND2/1(u1), AND1/1(u1)
  Data Type Conversion3/1 -> Mux/3
  AND2/1(y) -> Shift Arithmetic/1
  Shift Arithmetic/1 -> Data Type Conversion3/1
  Data Type Conversion4/1 -> Mux/1
  [boIgnition] -> Data Type Conversion4/1
  Shift Arithmetic1/1 -> Add/2
  Product8/1 -> Add/3
  Product1/1 -> Add/4
  Product2/1 -> Add/5
  Product3/1 -> Add/6
  Product4/1 -> Add/7
  Product5/1 -> Add/8
  Product6/1 -> Add/9
  Product7/1 -> Add/10
  Data Type Conversion5/1 -> Product8/1
  Data Type Conversion6/1 -> Product1/1
  Data Type Conversion7/1 -> Product2/1
  Data Type Conversion8/1 -> Product3/1
  Data Type Conversion9/1 -> Product4/1
  Data Type Conversion10/1 -> Product5/1
  Data Type Conversion11/1 -> Product6/1
  Data Type Conversion12/1 -> Product7/1
  Constant5/1 -> Product8/2
  Constant6/1 -> Product1/2
  Constant8/1 -> Product2/2
  Constant9/1 -> Product3/2
  Constant10/1 -> Product4/2
  Constant11/1 -> Product5/2
  Constant12/1 -> Product6/2
  Constant13/1 -> Product7/2
  Add/1 -> out_OUT_PCAN.Tx_Acc.Lin_Sts.BatteryVoltage/1
  Constant14/1 -> out_OUT_PCAN.Tx_Acc.Lin_Sts.MessageEnable/1
  Data Type Conversion13/1 -> out_OUT_PCAN.Tx_Acc.Lin_Sts.Button_KL15/1

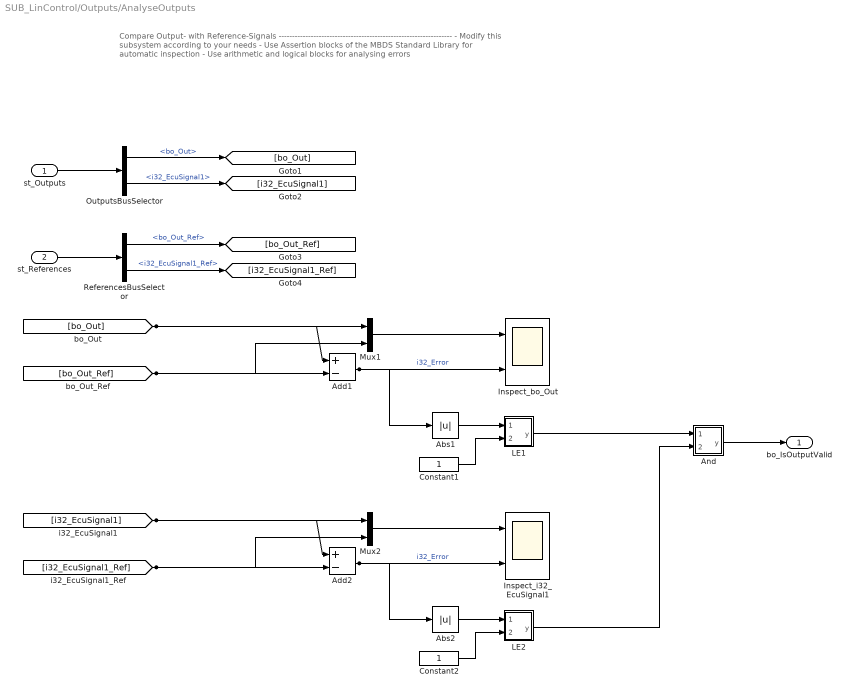
== system SUB_LinControl/Outputs/AnalyseOutputs ==
  note: Compare Output- with Reference-Signals
      | -----------------------------------------------------------------
      | - Modify this subsystem according to your needs
      | -  Use Assertion blocks of the MBDS Standard Library for automatic inspection
      | - Use arithmetic and logical blocks for analysing errors
  st_Outputs : Inport  InitFcn=|
      | try
      |    MBDS_BlockCallback('Update', gcb);
      | end
  st_References : Inport  InitFcn=|  Port=2
      | try
      |    MBDS_BlockCallback('Update', gcb);
      | end
  Abs1 : Abs  InitFcn=|  OutDataTypeStr=Inherit: Inherit via back propagation
      | if(exist('MBDS_BlockCallback', 'file'))
      |    MBDS_BlockCallback('Update', gcb);  
      | end
      settings: AttributesFormatString=Saturate: %<SaturateOnIntegerOverflow>
  Abs2 : Abs  InitFcn=|  OutDataTypeStr=Inherit: Inherit via back propagation
      | if(exist('MBDS_BlockCallback', 'file'))
      |    MBDS_BlockCallback('Update', gcb);  
      | end
      settings: AttributesFormatString=Saturate: %<SaturateOnIntegerOverflow>
  Add1 : Sum  InitFcn=|  Inputs=+-  OutDataTypeStr=int32  SaturateOnIntegerOverflow=on  InputSameDT=on
      | if(exist('MBDS_BlockCallback', 'file'))
      |    MBDS_BlockCallback('Update', gcb);  
      | end
      settings: AttributesFormatString=Saturate: %<SaturateOnIntegerOverflow>
  Add2 : Sum  InitFcn=|  Inputs=+-  OutDataTypeStr=int32  SaturateOnIntegerOverflow=on  InputSameDT=on
      | if(exist('MBDS_BlockCallback', 'file'))
      |    MBDS_BlockCallback('Update', gcb);  
      | end
      settings: AttributesFormatString=Saturate: %<SaturateOnIntegerOverflow>
  And : Subsystem  InitFcn=|  mask(AND){MBDS_LibraryBlock=on, BitwiseMode=off, Inputs=2, UseBitMask=off, BitMask='A7', OutDataTypeStr=Inherit: Inherit via back propagation, MBDS_BlockVersion=08.20.02}
      | if(exist('MBDS_BlockCallback', 'file'))
      |    MBDS_BlockCallback('Update', gcb);
      | end
      mask prompts: MBDS_LibraryBlock "MBDS library block"; BitwiseMode "Use 'bitwise' mode"; Inputs "Number of input ports:"; UseBitMask "Use bit mask"; BitMask "Bit mask:"; OutDataTypeStr "Output data type:"; MBDS_BlockVersion "Version:"
      mask help: Logical or bitwise AND operator. For multiple inputs, operators are applied across the inputs. For a single input, operators are applied across the input vector. In bitwise mode a bit mask can be applied onto single input signals.
      mask init: same as SUB_LinControl/Model/SUB_LinControl_/AND1
      mask Help: eval(['open([workdir(''library_dir:''),''\Blockset\help\'',get_param(gcb,''MaskType''),''.html''])'])
      mask Callback BitwiseMode:
      | if(exist('MBDS_BlockCallback', 'file'))
      |    MBDS_BlockCallback('BitwiseMode', gcb);
      | end
      mask Callback Inputs:
      | if(exist('MBDS_BlockCallback', 'file'))
      |    MBDS_BlockCallback('Inputs', gcb);
      | end
      mask Callback UseBitMask:
      | if(exist('MBDS_BlockCallback', 'file'))
      |    MBDS_BlockCallback('UseBitMask', gcb);
      | end
      mask Callback BitMask:
      | if(exist('MBDS_BlockCallback', 'file'))
      |    MBDS_BlockCallback('BitMask', gcb);
      | end
      mask TypeOptions OutDataTypeStr: Inherit: Inherit via back propagation | int8 | uint8 | int16 | uint16 | int32 | uint32 | boolean
      mask Callback OutDataTypeStr:
      | % Adopt Value
      | if(exist('MBDS_BlockCallback', 'file'))
      |    MBDS_BlockCallback('OutDataTypeStr', gcb);
      | end
      mask DialogControl ParameterTabVar0 Prompt: Main
      mask DialogControl ParameterTabVar01 Prompt: Signal Attributes
      mask DialogControl ParameterTabVar012 Prompt: Version
      mask Display:
      | % Show icon or block text
      | if(UseBitMask)
      |    if(isnumeric(BitMask))
      |       BitMaskString = ['0x',dec2hex(floor(BitMask))];
      |    elseif(ischar(BitMask))
      |       BitMaskString = ['0x',upper(BitMask)];
      |    else
      |       BitMaskString = '???';
      |    end
      |    disp(sprintf(['AND\n', BitMaskString]))
      | else
      |    disp('AND')
      | end
  Constant1 : Constant  InitFcn=|  OutDataTypeStr=Inherit: Inherit via back propagation
      | if(exist('MBDS_BlockCallback', 'file'))
      |    MBDS_BlockCallback('Update', gcb);  
      | end
  Constant2 : Constant  InitFcn=|  OutDataTypeStr=Inherit: Inherit via back propagation
      | if(exist('MBDS_BlockCallback', 'file'))
      |    MBDS_BlockCallback('Update', gcb);  
      | end
  Inspect_bo_Out : Scope  NumInputPorts=2
  Inspect_i32_EcuSignal1 : Scope  NumInputPorts=2
  LE1 : Subsystem  InitFcn=|  mask(LE){MBDS_LibraryBlock=on, InputSameDT=on, MBDS_BlockVersion=05.20}
      | if(exist('MBDS_BlockCallback', 'file'))
      |    MBDS_BlockCallback('Update', gcb);
      | end
      mask prompts: MBDS_LibraryBlock "MBDS library block"; InputSameDT "Require all inputs to have the same data type"; MBDS_BlockVersion "Block version:"
      mask help: The block compares if the first input signal is lower than or equal to the second input signal.
      mask init: same as SUB_LinControl/Model/SUB_LinControl_/AND1
      mask Help: eval(['open([workdir(''library_dir:''),''\Blockset\help\'',get_param(gcb,''MaskType''),''.html''])'])
      mask Callback InputSameDT:
      | % Adopt value
      | if(exist('MBDS_BlockCallback', 'file'))
      |    MBDS_BlockCallback('InputSameDT', gcb);
      | end
      mask DialogControl ParameterTabVar0 Prompt: Signal Attributes
      mask DialogControl ParameterTabVar01 Prompt: Version
      mask Display:
      | % Show icon or block text
      | if(exist('MBDS_BlockCallback', 'file'))
      |    image(imread('LE.tif','tif'),[0.33,0.33,0.37,0.37])
      |    disp('')
      | else
      |    disp(sprintf('<='));
      | end
  LE2 : Subsystem  InitFcn=|  mask(LE){MBDS_LibraryBlock=on, InputSameDT=on, MBDS_BlockVersion=05.20}
      | if(exist('MBDS_BlockCallback', 'file'))
      |    MBDS_BlockCallback('Update', gcb);
      | end
      mask prompts: MBDS_LibraryBlock "MBDS library block"; InputSameDT "Require all inputs to have the same data type"; MBDS_BlockVersion "Block version:"
      mask help: The block compares if the first input signal is lower than or equal to the second input signal.
      mask init: same as SUB_LinControl/Model/SUB_LinControl_/AND1
      mask Help: eval(['open([workdir(''library_dir:''),''\Blockset\help\'',get_param(gcb,''MaskType''),''.html''])'])
      mask Callback InputSameDT:
      | % Adopt value
      | if(exist('MBDS_BlockCallback', 'file'))
      |    MBDS_BlockCallback('InputSameDT', gcb);
      | end
      mask DialogControl ParameterTabVar0 Prompt: Signal Attributes
      mask DialogControl ParameterTabVar01 Prompt: Version
      mask Display:
      | % Show icon or block text
      | if(exist('MBDS_BlockCallback', 'file'))
      |    image(imread('LE.tif','tif'),[0.33,0.33,0.37,0.37])
      |    disp('')
      | else
      |    disp(sprintf('<='));
      | end
  Mux1 : Mux  InitFcn=|  Inputs=2
      | try
      |    MBDS_BlockCallback('Update', gcb);
      | end
  Mux2 : Mux  InitFcn=|  Inputs=2
      | try
      |    MBDS_BlockCallback('Update', gcb);
      | end
  OutputsBusSelector : BusSelector  InitFcn=|  OutputSignals=st_Outputs.bo_Out,i32_EcuSignal1
      | try
      |    MBDS_BlockCallback('Update', gcb);
      | end
  ReferencesBusSelector : BusSelector  InitFcn=|  OutputSignals=st_Outputs.bo_Out_Ref,i32_EcuSignal1_Ref
      | try
      |    MBDS_BlockCallback('Update', gcb);
      | end
  bo_IsOutputValid : Outport  InitFcn=|  PortDimensions=1
      | try
      |    MBDS_BlockCallback('Update', gcb);
      | end
  wires:
  st_Outputs/1 -> OutputsBusSelector/1
  OutputsBusSelector/1 -> [bo_Out]  "<bo_Out>"
  OutputsBusSelector/2 -> [i32_EcuSignal1]  "<i32_EcuSignal1>"
  st_References/1 -> ReferencesBusSelector/1
  ReferencesBusSelector/1 -> [bo_Out_Ref]  "<bo_Out_Ref>"
  ReferencesBusSelector/2 -> [i32_EcuSignal1_Ref]  "<i32_EcuSignal1_Ref>"
  [bo_Out_Ref] -> Add1/2, Mux1/2
  [bo_Out] -> Add1/1, Mux1/1
  Mux1/1 -> Inspect_bo_Out/1
  Add1/1 -> Abs1/1, Inspect_bo_Out/2  "i32_Error"
  Abs1/1 -> LE1/1(u1)
  Constant1/1 -> LE1/2(u2)
  [i32_EcuSignal1_Ref] -> Add2/2, Mux2/2
  [i32_EcuSignal1] -> Add2/1, Mux2/1
  Mux2/1 -> Inspect_i32_EcuSignal1/1
  Add2/1 -> Abs2/1, Inspect_i32_EcuSignal1/2  "i32_Error"
  Abs2/1 -> LE2/1(u1)
  Constant2/1 -> LE2/2(u2)
  And/1(y) -> bo_IsOutputValid/1
  LE1/1(y) -> And/1(u1)
  LE2/1(y) -> And/2(u2)

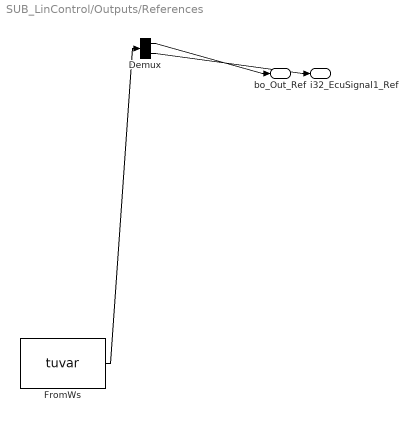
== system SUB_LinControl/Outputs/References ==
  Demux : Demux  Tag=STV Demux  Outputs=2
  FromWs : FromWorkspace  Tag=STV FromWs  VariableName=tuvar
      SigBuilderData=|
      | dataSet.timeRange = [0 10]
      | dataSet.name = 'TC1'
      | sbobj.Name = 'Signal Builder'
      | sbobj.Groups.Name = 'TC1'
      | sbobj.Groups.Signals(1).Name = 'bo_Out_Ref'
      | sbobj.Groups.Signals(1).XData = [0 1 2 3 4 4 5 6 6 7 8 9 10]
      | sbobj.Groups.Signals(1).YData = [0 0 0 0 0 1 1 1 0 0 0 0 0]
      | sbobj.Groups.Signals(2).Name = 'i32_EcuSignal1_Ref'
      | sbobj.Groups.Signals(2).XData = [0 1 2 3 4 5 6 7 8 9 10]
      | sbobj.Groups.Signals(2).YData = [1 1 1 1 1 1 1 1 1 1 1]
  bo_Out_Ref : Outport  Tag=STV Outport
  i32_EcuSignal1_Ref : Outport  Tag=STV Outport  Port=2
  wires:
  FromWs/1 -> Demux/1
  Demux/1 -> bo_Out_Ref/1
  Demux/2 -> i32_EcuSignal1_Ref/1

== system SUB_LinControl/Stimuli/Stimuli ==
  Demux : Demux  Tag=STV Demux  Outputs=1
  FromWs : FromWorkspace  Tag=STV FromWs  VariableName=tuvar
      SigBuilderData=|
      | dataSet.timeRange = [0 10]
      | dataSet.name = 'TC1'
      | sbobj.Name = 'Signal Builder'
      | sbobj.Groups.Name = 'TC1'
      | sbobj.Groups.Signals.Name = 'bo_In'
      | sbobj.Groups.Signals.XData = [0 1 2 3 4 4 5 6 6 7 8 9 10]
      | sbobj.Groups.Signals.YData = [0 0 0 0 0 1 1 1 0 0 0 0 0]
  bo_In : Outport  Tag=STV Outport
  wires:
  FromWs/1 -> Demux/1
  Demux/1 -> bo_In/1

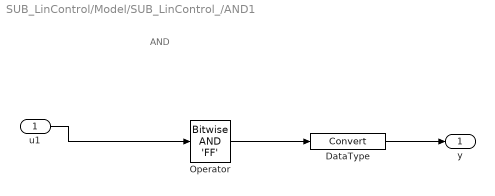
== system SUB_LinControl/Model/SUB_LinControl_/AND1 ==
  note: AND
  u1 : Inport
  DataType : DataTypeConversion
  Operator : simulink/Logic and Bit Operations/Bitwise Operator  logicop=AND  UseBitMask=on  BitMask='FF'  BitMaskRealWorld=Stored Integer
  y : Outport
  wires:
  Operator/1 -> DataType/1
  u1/1 -> Operator/1
  DataType/1 -> y/1

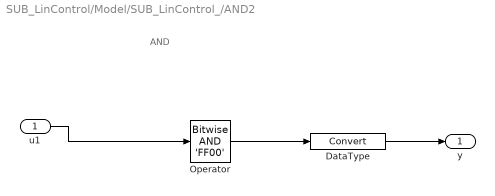
== system SUB_LinControl/Model/SUB_LinControl_/AND2 ==
  note: AND
  u1 : Inport
  DataType : DataTypeConversion
  Operator : simulink/Logic and Bit Operations/Bitwise Operator  logicop=AND  UseBitMask=on  BitMask='FF00'  BitMaskRealWorld=Stored Integer
  y : Outport
  wires:
  Operator/1 -> DataType/1
  u1/1 -> Operator/1
  DataType/1 -> y/1

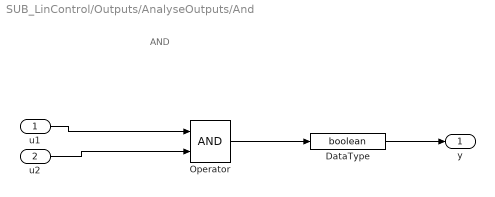
== system SUB_LinControl/Outputs/AnalyseOutputs/And ==
  note: AND
  u1 : Inport  OutDataTypeStr=boolean
  u2 : Inport  Port=2  OutDataTypeStr=boolean
  DataType : DataTypeConversion  OutDataTypeStr=boolean
  Operator : Logic  AllPortsSameDT=off  OutDataTypeStr=boolean
  y : Outport
  wires:
  Operator/1 -> DataType/1
  u1/1 -> Operator/1
  u2/1 -> Operator/2
  DataType/1 -> y/1

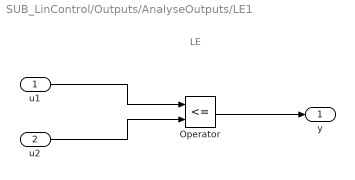
== system SUB_LinControl/Outputs/AnalyseOutputs/LE1 ==
  note: LE
  u1 : Inport
  u2 : Inport  Port=2
  Operator : RelationalOperator  Operator=<=  OutDataTypeStr=boolean  RndMeth=Nearest  InputSameDT=on
  y : Outport
  wires:
  Operator/1 -> y/1
  u2/1 -> Operator/2
  u1/1 -> Operator/1

== system SUB_LinControl/Outputs/AnalyseOutputs/LE2 ==
  note: LE
  u1 : Inport
  u2 : Inport  Port=2
  Operator : RelationalOperator  Operator=<=  OutDataTypeStr=boolean  RndMeth=Nearest  InputSameDT=on
  y : Outport
  wires:
  Operator/1 -> y/1
  u2/1 -> Operator/2
  u1/1 -> Operator/1
